simulink model "DynamiqueSphere"  (R2018b)
settings: Solver=VariableStepAuto  StartTime=0.0  StopTime=10.0  RelTol=1e-3
values from neighbouring files (symbols this model uses):
  g = 9.81    [Modele.m]
undefined symbols (not defined in the file or in its folder): JS, mS, rS
libraries: dspsrcs4 x2
settings Model: Creator=Vincent  LastModifiedBy=Vincent

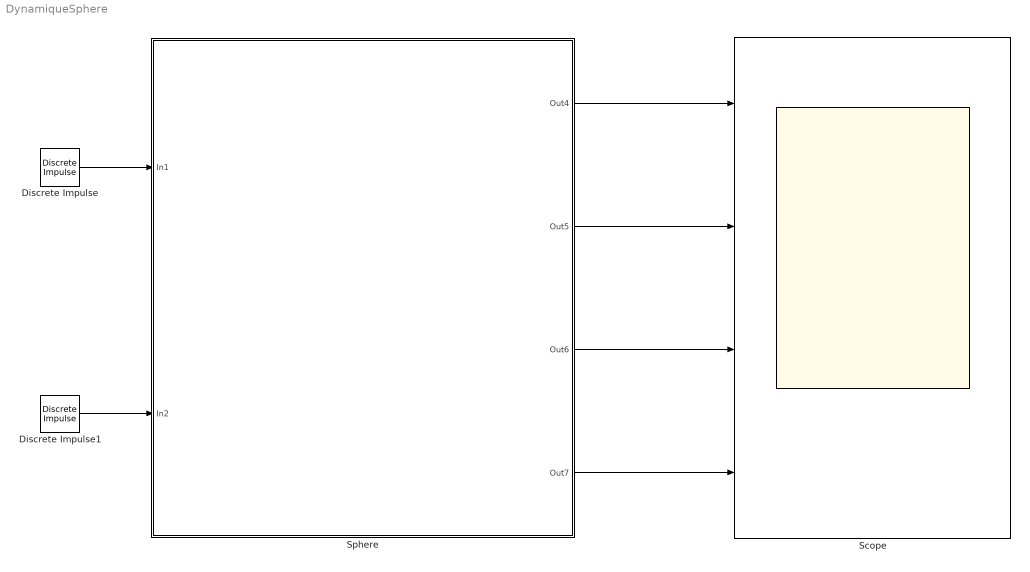
== system DynamiqueSphere ==
  Discrete Impulse : dspsrcs4/Discrete  Impulse  Delay=0  SampleTime=1  FrameSample=1  OutputFrames=off  dataType=double  isSigned=on  wordLen=16  udDataType=sfix(16)  fracBitsMode=Best precision  numFracBits=15  OutDataTypeStr=double  LastOutDataTypeStr=double
  Discrete Impulse1 : dspsrcs4/Discrete  Impulse  Delay=0  SampleTime=1  FrameSample=1  OutputFrames=off  dataType=double  isSigned=on  wordLen=16  udDataType=sfix(16)  fracBitsMode=Best precision  numFracBits=15  OutDataTypeStr=double  LastOutDataTypeStr=double
  Scope : Scope  NumInputPorts=4
  Sphere : Subsystem
  wires:
  Discrete Impulse1/1 -> Sphere/2(In2)
  Discrete Impulse/1 -> Sphere/1(In1)
  Sphere/1(Out4) -> Scope/1
  Sphere/2(Out5) -> Scope/2
  Sphere/3(Out6) -> Scope/3
  Sphere/4(Out7) -> Scope/4

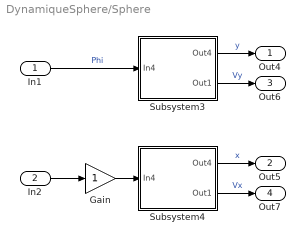
== system DynamiqueSphere/Sphere ==
  In1 : Inport
  In2 : Inport  Port=2
  Gain : Gain
  Subsystem3 : Subsystem
  Subsystem4 : Subsystem
  Out4 : Outport
  Out5 : Outport  Port=2
  Out6 : Outport  Port=3
  Out7 : Outport  Port=4
  wires:
  Subsystem3/2(Out1) -> Out6/1  "Vy"
  Subsystem4/1(Out4) -> Out5/1  "x"
  Subsystem3/1(Out4) -> Out4/1  "y"
  In2/1 -> Gain/1
  Subsystem4/2(Out1) -> Out7/1  "Vx"
  Gain/1 -> Subsystem4/1(In4)
  In1/1 -> Subsystem3/1(In4)  "Phi"

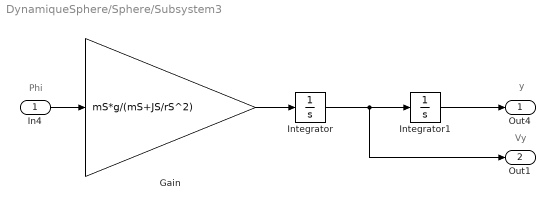
== system DynamiqueSphere/Sphere/Subsystem3 ==
  note: y
  note: Vy
  note: Phi
  In4 : Inport  Tag=Theta
  Gain : Gain  Gain=mS*g/(mS+JS/rS^2)
  Integrator : Integrator
  Integrator1 : Integrator
  Out4 : Outport
  Out1 : Outport  Port=2
  wires:
  Gain/1 -> Integrator/1
  In4/1 -> Gain/1
  Integrator1/1 -> Out4/1
  Integrator/1 -> Out1/1, Integrator1/1

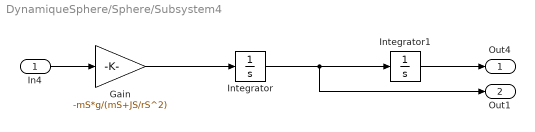
== system DynamiqueSphere/Sphere/Subsystem4 ==
  In4 : Inport  Tag=Theta
  Gain : Gain  Gain=-mS*g/(mS+JS/rS^2)
  Integrator : Integrator
  Integrator1 : Integrator
  Out4 : Outport
  Out1 : Outport  Port=2
  wires:
  Gain/1 -> Integrator/1
  In4/1 -> Gain/1
  Integrator1/1 -> Out4/1
  Integrator/1 -> Out1/1, Integrator1/1
